simulink model "lidar_output_simulation"  (R2019b)
settings: Solver=VariableStepAuto  StartTime=0.0  StopTime=5  RelTol=1e-3
undefined symbols (not defined in the file): __PRM__SERIALIZED__DATA__, SubsystemReferenceBlock
settings Model: Creator=jingg  LastModifiedBy=jingg

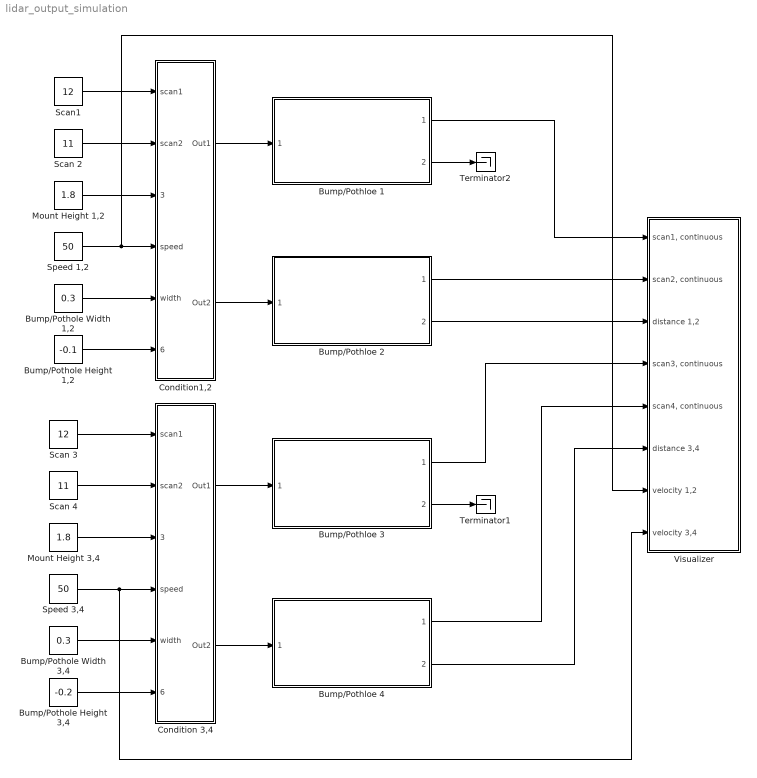
== system lidar_output_simulation ==
  Bump/Pothloe {1..4} (4 alike) : Subsystem  BlockKeywords=__PRM__SERIALIZED__DATA__:SubsystemReferenceBlock  ReferencedSubsystem=bump_mdl
  Bump/Pothole Height 1,2 : Constant  Value=-0.1
  Bump/Pothole Height 3,4 : Constant  Value=-0.2
  Bump/Pothole Width 1,2 : Constant  Value=0.3
  Bump/Pothole Width 3,4 : Constant  Value=0.3
  Condition 3,4 : Subsystem
  Condition1,2 : Subsystem
  Mount Height 1,2 : Constant  Value=1.8
  Mount Height 3,4 : Constant  Value=1.8
  Scan 2 : Constant  Value=11  SampleTime=11
  Scan 3 : Constant  Value=12
  Scan 4 : Constant  Value=11  SampleTime=11
  Scan1 : Constant  Value=12
  Speed 1,2 : Constant  Value=50
  Speed 3,4 : Constant  Value=50
  Terminator1 : Terminator
  Terminator2 : Terminator
  Visualizer : Subsystem
  wires:
  Scan1/1 -> Condition1,2/1(scan1)
  Scan 2/1 -> Condition1,2/2(scan2)
  Mount Height 1,2/1 -> Condition1,2/3(mount_h)
  Speed 1,2/1 -> Visualizer/7(velocity 1,2), Condition1,2/4(speed)
  Bump/Pothole Width 1,2/1 -> Condition1,2/5(width)
  Bump/Pothole Height 1,2/1 -> Condition1,2/6(height)
  Condition1,2/1(Out1) -> Bump/Pothloe 1/1
  Condition1,2/2(Out2) -> Bump/Pothloe 2/1
  Condition 3,4/1(Out1) -> Bump/Pothloe 3/1
  Condition 3,4/2(Out2) -> Bump/Pothloe 4/1
  Scan 3/1 -> Condition 3,4/1(scan1)
  Bump/Pothole Height 3,4/1 -> Condition 3,4/6(height)
  Bump/Pothole Width 3,4/1 -> Condition 3,4/5(width)
  Speed 3,4/1 -> Visualizer/8(velocity 3,4), Condition 3,4/4(speed)
  Mount Height 3,4/1 -> Condition 3,4/3(mount_h)
  Scan 4/1 -> Condition 3,4/2(scan2)
  Bump/Pothloe 1/2 -> Terminator2/1
  Bump/Pothloe 3/2 -> Terminator1/1
  Bump/Pothloe 1/1 -> Visualizer/1("scan1, continuous")
  Bump/Pothloe 2/1 -> Visualizer/2("scan2, continuous")
  Bump/Pothloe 2/2 -> Visualizer/3(distance 1,2)
  Bump/Pothloe 3/1 -> Visualizer/4("scan3, continuous")
  Bump/Pothloe 4/1 -> Visualizer/5("scan4, continuous")
  Bump/Pothloe 4/2 -> Visualizer/6(distance 3,4)

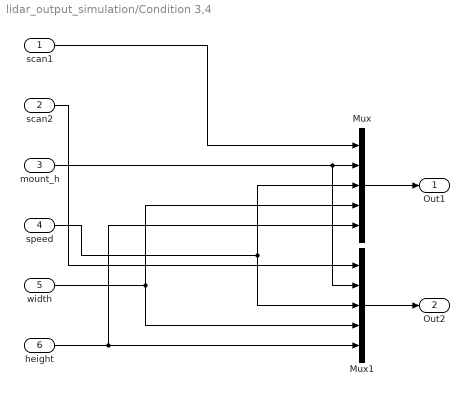
== system lidar_output_simulation/Condition 3,4 ==
  scan1 : Inport
  scan2 : Inport  Port=2
  mount_h : Inport  Port=3
  speed : Inport  Port=4
  width : Inport  Port=5
  height : Inport  Port=6
  Mux : Mux  Inputs=5
  Mux1 : Mux  Inputs=5
  Out1 : Outport
  Out2 : Outport  Port=2
  wires:
  scan2/1 -> Mux1/1
  mount_h/1 -> Mux/2, Mux1/2
  width/1 -> Mux/4, Mux1/4
  height/1 -> Mux/5, Mux1/5
  scan1/1 -> Mux/1
  speed/1 -> Mux/3, Mux1/3
  Mux/1 -> Out1/1
  Mux1/1 -> Out2/1

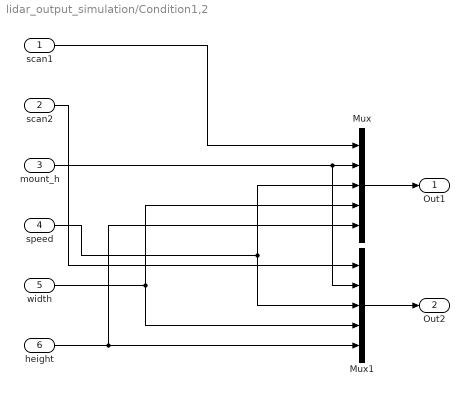
== system lidar_output_simulation/Condition1,2 ==
  scan1 : Inport
  scan2 : Inport  Port=2
  mount_h : Inport  Port=3
  speed : Inport  Port=4
  width : Inport  Port=5
  height : Inport  Port=6
  Mux : Mux  Inputs=5
  Mux1 : Mux  Inputs=5
  Out1 : Outport
  Out2 : Outport  Port=2
  wires:
  Mux1/1 -> Out2/1
  Mux/1 -> Out1/1
  speed/1 -> Mux1/3, Mux/3
  scan1/1 -> Mux/1
  height/1 -> Mux1/5, Mux/5
  width/1 -> Mux1/4, Mux/4
  mount_h/1 -> Mux1/2, Mux/2
  scan2/1 -> Mux1/1

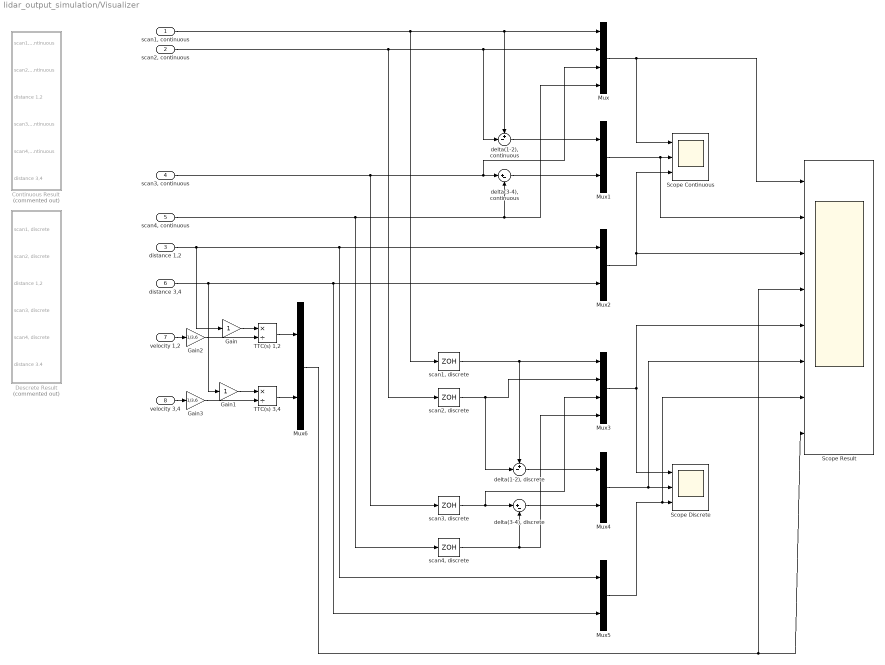
== system lidar_output_simulation/Visualizer ==
  "scan1, continuous" : Inport
  "scan2, continuous" : Inport  Port=2
  distance 1,2 : Inport  Port=3
  "scan3, continuous" : Inport  Port=4
  "scan4, continuous" : Inport  Port=5
  distance 3,4 : Inport  Port=6
  velocity 1,2 : Inport  Port=7
  velocity 3,4 : Inport  Port=8
  Continuous Result : Subsystem  Commented=on
  Descrete Result : Subsystem  Commented=on
  Gain : Gain
  Gain1 : Gain
  Gain2 : Gain  Gain=1/3.6
  Gain3 : Gain  Gain=1/3.6
  Mux : Mux
  Mux{1..2,4..6} (5 alike) : Mux  Inputs=2
  Mux3 : Mux
  Scope Continuous : Scope  NumInputPorts=3
  Scope Discrete : Scope  NumInputPorts=3
  Scope Result : Scope  NumInputPorts=8
  TTC(s) 1,2 : Product  Inputs=*/
  TTC(s) 3,4 : Product  Inputs=*/
  "delta(1-2), continuous" : Sum  Inputs=+-|
  "delta(1-2), discrete" : Sum  Inputs=+-|
  "delta(3-4), continuous" : Sum  Inputs=|+-
  "delta(3-4), discrete" : Sum  Inputs=|+-
  "scan1, discrete" : ZeroOrderHold  SampleTime=0.1
  "scan2, discrete" : ZeroOrderHold  SampleTime=0.1
  "scan3, discrete" : ZeroOrderHold  SampleTime=0.1
  "scan4, discrete" : ZeroOrderHold  SampleTime=0.1
  wires:
  "scan2, continuous"/1 -> "scan2, discrete"/1, "delta(1-2), continuous"/2, Mux/2
  Mux1/1 -> Scope Result/2, Scope Continuous/2
  "scan3, continuous"/1 -> "scan3, discrete"/1, Mux/3, "delta(3-4), continuous"/1
  "delta(3-4), continuous"/1 -> Mux1/2
  "delta(1-2), continuous"/1 -> Mux1/1
  Mux2/1 -> Scope Continuous/3, Scope Result/3
  Mux/1 -> Scope Result/1, Scope Continuous/1
  "scan4, continuous"/1 -> "scan4, discrete"/1, Mux/4, "delta(3-4), continuous"/2
  "scan2, discrete"/1 -> "delta(1-2), discrete"/2, Mux3/2
  Mux4/1 -> Scope Result/6, Scope Discrete/2
  "delta(3-4), discrete"/1 -> Mux4/2
  "scan1, continuous"/1 -> "scan1, discrete"/1, "delta(1-2), continuous"/1, Mux/1
  Mux3/1 -> Scope Result/5, Scope Discrete/1
  Mux5/1 -> Scope Result/7, Scope Discrete/3
  "delta(1-2), discrete"/1 -> Mux4/1
  "scan1, discrete"/1 -> "delta(1-2), discrete"/1, Mux3/1
  "scan3, discrete"/1 -> Mux3/3, "delta(3-4), discrete"/1
  "scan4, discrete"/1 -> Mux3/4, "delta(3-4), discrete"/2
  distance 1,2/1 -> Gain/1, Mux5/1, Mux2/1
  distance 3,4/1 -> Gain1/1, Mux5/2, Mux2/2
  velocity 1,2/1 -> Gain2/1
  velocity 3,4/1 -> Gain3/1
  Gain/1 -> TTC(s) 1,2/1
  Gain1/1 -> TTC(s) 3,4/1
  TTC(s) 1,2/1 -> Mux6/1
  TTC(s) 3,4/1 -> Mux6/2
  Mux6/1 -> Scope Result/4, Scope Result/8
  Gain2/1 -> TTC(s) 1,2/2
  Gain3/1 -> TTC(s) 3,4/2

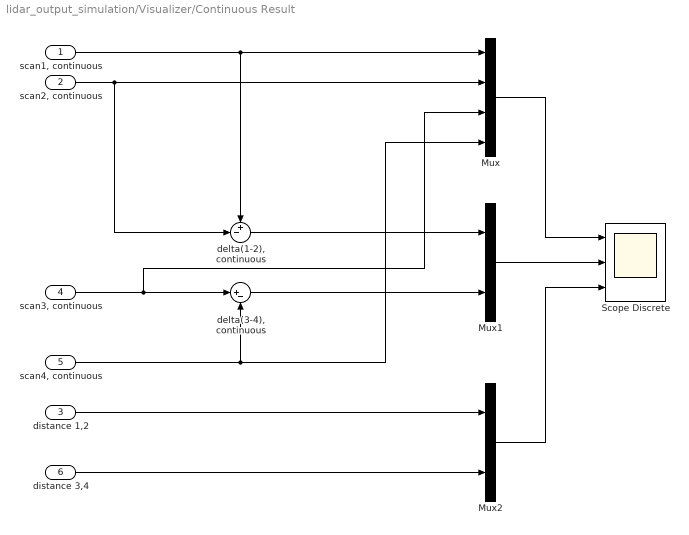
== system lidar_output_simulation/Visualizer/Continuous Result ==
  "scan1, continuous" : Inport
  "scan2, continuous" : Inport  Port=2
  distance 1,2 : Inport  Port=3
  "scan3, continuous" : Inport  Port=4
  "scan4, continuous" : Inport  Port=5
  distance 3,4 : Inport  Port=6
  Mux : Mux
  Mux1 : Mux  Inputs=2
  Mux2 : Mux  Inputs=2
  Scope Discrete : Scope  NumInputPorts=3
  "delta(1-2), continuous" : Sum  Inputs=+-|
  "delta(3-4), continuous" : Sum  Inputs=|+-
  wires:
  "delta(3-4), continuous"/1 -> Mux1/2
  "delta(1-2), continuous"/1 -> Mux1/1
  "scan4, continuous"/1 -> Mux/4, "delta(3-4), continuous"/2
  distance 3,4/1 -> Mux2/2
  "scan3, continuous"/1 -> Mux/3, "delta(3-4), continuous"/1
  "scan2, continuous"/1 -> "delta(1-2), continuous"/2, Mux/2
  "scan1, continuous"/1 -> "delta(1-2), continuous"/1, Mux/1
  distance 1,2/1 -> Mux2/1
  Mux/1 -> Scope Discrete/1
  Mux1/1 -> Scope Discrete/2
  Mux2/1 -> Scope Discrete/3

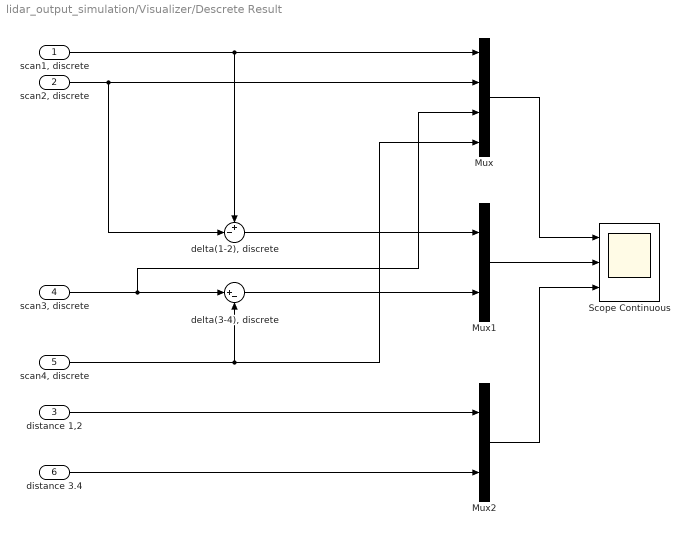
== system lidar_output_simulation/Visualizer/Descrete Result ==
  "scan1, discrete" : Inport
  "scan2, discrete" : Inport  Port=2
  distance 1,2 : Inport  Port=3
  "scan3, discrete" : Inport  Port=4
  "scan4, discrete" : Inport  Port=5
  distance 3.4 : Inport  Port=6
  Mux : Mux
  Mux1 : Mux  Inputs=2
  Mux2 : Mux  Inputs=2
  Scope Continuous : Scope  NumInputPorts=3
  "delta(1-2), discrete" : Sum  Inputs=+-|
  "delta(3-4), discrete" : Sum  Inputs=|+-
  wires:
  "scan2, discrete"/1 -> "delta(1-2), discrete"/2, Mux/2
  Mux1/1 -> Scope Continuous/2
  distance 3.4/1 -> Mux2/2
  "scan3, discrete"/1 -> Mux/3, "delta(3-4), discrete"/1
  "delta(3-4), discrete"/1 -> Mux1/2
  "delta(1-2), discrete"/1 -> Mux1/1
  Mux2/1 -> Scope Continuous/3
  Mux/1 -> Scope Continuous/1
  "scan1, discrete"/1 -> "delta(1-2), discrete"/1, Mux/1
  distance 1,2/1 -> Mux2/1
  "scan4, discrete"/1 -> Mux/4, "delta(3-4), discrete"/2
